simulink model "m4s"  (R2022a)
settings: Solver=VariableStepAuto  StartTime=0.0  StopTime=100  RelTol=1e-3
values from neighbouring files (symbols this model uses):
  delta_da = 0.2    [m1.m]    (also in m2.m = 0; m3.m = 0)
  delta_dt = 0    [m1.m]    (also in m2.m; m3.m)
  delta_dy = 0    [m1.m]    (also in m2.m; m3.m)
  rho = 0    [m1.m]    (also in m2.m = 1; m3.m = 1)
undefined symbols (not defined in the file or in its folder): wy
libraries: cstblocks x2, simulink x1
settings Model: Creator=apple  LastModifiedBy=apple

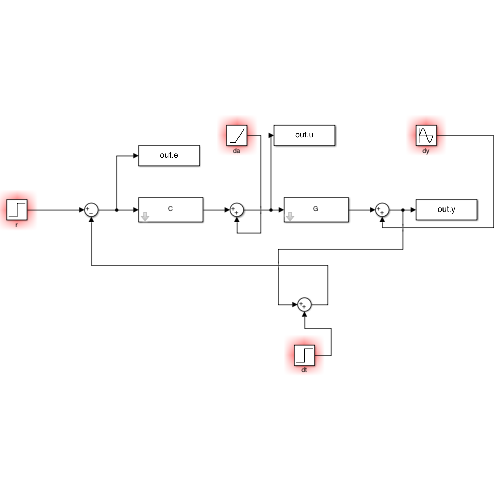
[thumbnail: Simulink's stored preview of the top-level diagram]
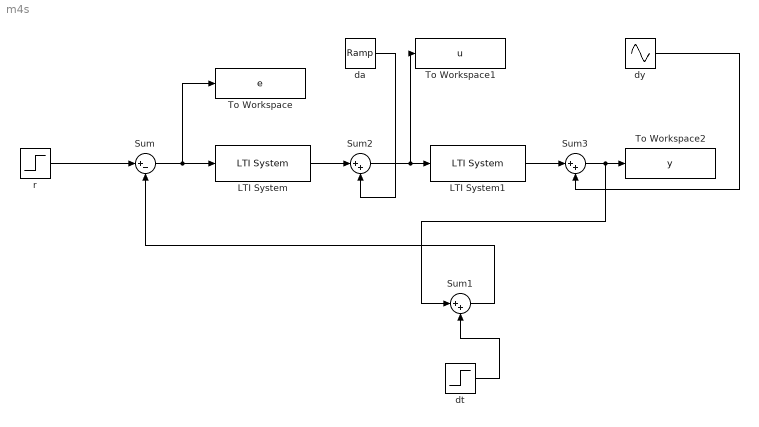
== system m4s ==
  LTI System : cstblocks/LTI System  sys=C  IC=[]
  LTI System1 : cstblocks/LTI System  sys=G  IC=[]
  Sum : Sum  Inputs=|+-
  Sum1 : Sum  Inputs=|++
  Sum2 : Sum  Inputs=|++
  Sum3 : Sum  Inputs=|++
  To Workspace : ToWorkspace  VariableName=e  SaveFormat=Timeseries  SampleTime=-1
  To Workspace1 : ToWorkspace  VariableName=u  SaveFormat=Timeseries  SampleTime=-1
  To Workspace2 : ToWorkspace  VariableName=y  SaveFormat=Timeseries  SampleTime=-1
  da : simulink/Sources/Ramp  slope=delta_da  start=0  InitialOutput=0
  dt : Step  Time=0  After=delta_dt  SampleTime=0
  dy : Sin  Amplitude=delta_dy  Frequency=wy  SampleTime=0
  r : Step  Time=0  After=rho  SampleTime=0
  wires:
  dt/1 -> Sum1/2
  da/1 -> Sum2/2
  Sum2/1 -> To Workspace1/1, LTI System1/1
  LTI System/1 -> Sum2/1
  dy/1 -> Sum3/2
  LTI System1/1 -> Sum3/1
  Sum3/1 -> Sum1/1, To Workspace2/1
  Sum1/1 -> Sum/2
  Sum/1 -> To Workspace/1, LTI System/1
  r/1 -> Sum/1
